simulink model "sim2DOFArmSynergyTemplate"  (R2017a)
settings: Solver=FixedStepAuto  StartTime=0.0  StopTime=6  RelTol=1e-3
undefined symbols (not defined in the file): alpha, armDynamics, get
libraries: vrlib x4, sldrtlib x1
settings Model: Creator=ricardog  LastModifiedBy=ricardog
settings SolverCC: AutoInsertRateTranBlk=on

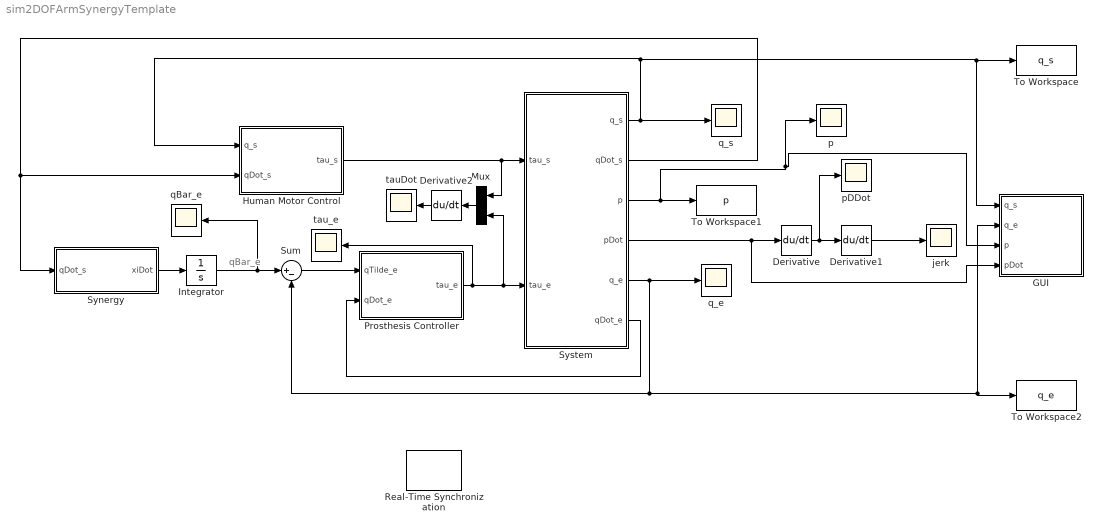
== system sim2DOFArmSynergyTemplate ==
  note: qBar_e
  Derivative : Derivative
  Derivative1 : Derivative
  Derivative2 : Derivative
  GUI : Subsystem
  Human Motor Control : Subsystem
  Integrator : Integrator  InitialCondition=get(armDynamics,'qInit_e')
  Mux : Mux  Inputs=2
  Prosthesis Controller : Subsystem
  Real-Time Synchronization : sldrtlib/Real-Time Synchronization  SampleTime=0.01  MaxMissedTicks=50  ShowMissedTicks=off  YieldWhenWaiting=off
  Sum : Sum  Inputs=|+-
  Synergy : Subsystem
  System : Subsystem
  To Workspace : ToWorkspace  VariableName=q_s  SampleTime=-1
  To Workspace1 : ToWorkspace  VariableName=p  SampleTime=-1
  To Workspace2 : ToWorkspace  VariableName=q_e  SampleTime=-1
  jerk : Scope
  p : Scope
  pDDot : Scope
  qBar_e : Scope
  q_e : Scope
  q_s : Scope
  tauDot : Scope
  tau_e : Scope
  wires:
  Human Motor Control/1(tau_s) -> Mux/1, System/1(tau_s)
  Prosthesis Controller/1(tau_e) -> Mux/2, System/2(tau_e), tau_e/1
  System/6(qDot_e) -> Prosthesis Controller/2(qDot_e)
  System/5(q_e) -> q_e/1, GUI/2(q_e), To Workspace2/1, Sum/2
  Sum/1 -> Prosthesis Controller/1(qTilde_e)
  Synergy/1(xiDot) -> Integrator/1
  Integrator/1 -> qBar_e/1, Sum/1
  System/3(p) -> To Workspace1/1, GUI/3(p), p/1
  System/4(pDot) -> GUI/4(pDot), Derivative/1
  Derivative/1 -> pDDot/1, Derivative1/1
  Derivative1/1 -> jerk/1
  System/2(qDot_s) -> Human Motor Control/2(qDot_s), Synergy/1(qDot_s)
  Derivative2/1 -> tauDot/1
  Mux/1 -> Derivative2/1
  System/1(q_s) -> GUI/1(q_s), To Workspace/1, Human Motor Control/1(q_s), q_s/1

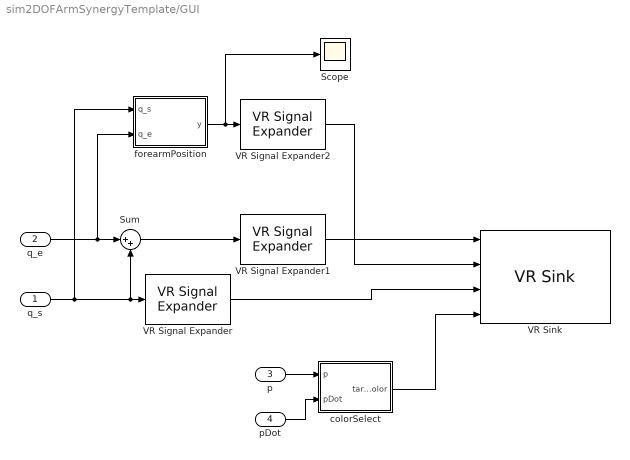
== system sim2DOFArmSynergyTemplate/GUI ==
  q_s : Inport
  q_e : Inport  Port=2
  p : Inport  Port=3
  pDot : Inport  Port=4
  Scope : Scope
  Sum : Sum  Inputs=|++
  VR Signal Expander : vrlib/VR Signal Expander  outwidth=4  outidx=[4]
      settings: SourceProductName=Simulink 3D Animation  SourceProductBaseCode=VR
  VR Signal Expander1 : vrlib/VR Signal Expander  outwidth=4  outidx=[4]
      settings: SourceProductName=Simulink 3D Animation  SourceProductBaseCode=VR
  VR Signal Expander2 : vrlib/VR Signal Expander  outwidth=3  outidx=[1 2]
      settings: SourceProductName=Simulink 3D Animation  SourceProductBaseCode=VR
  VR Sink : vrlib/VR Sink  InstantiateOnLoad=on  SampleTime=0.1  ViewEnable=on  RemoteChange=off  RemoteView=off  FieldsWritten=Forearm.rotation.4.1.1.double#Forearm.translation.3.1.1.double#UpperArm.rotation.4.1.1.double#EndTarget_material.diffuseColor.3.1.1.double  WorldFileName=C:\Users\ricardog\Documents\Workspace\HRSC_FW\GUI\armTargetsGUI.wrl  AutoView=on  VideoDimensions=[]  AllowVariableSize=off  FigureProperties="{'Position', 'Name', 'Viewpoint', 'CameraBound', 'CameraDirection', 'CameraPosition', 'CameraUpVector', 'ZoomFactor', 'Antialiasing', 'Headlight', 'Lighting', 'NavPanel', 'Sound', 'StatusBar', 'Stereo3D', 'Stereo3DCameraOffset', 'Stereo3DHIT', 'ToolBar', 'Textures', 'Transparency', 'Triad', 'Wireframe', 'NavZones', 'NavMode', 'NavSpeed', 'CaptureFileFormat', 'CaptureFileName', 'Record2DCompressMethod', 'Record2DCompressQuality', 'Record2D', 'Record2DFileName', 'Record2DFPS'; [5.8000000000000007e+00   9.1799999999999955e+01   6.8880000000000007e+02   4.7160000000000002e+02], '', 'Side view', 'on', [0.0000000000000000e+00   0.0000000000000000e+00  -1.0000000000000000e+00], [0.0000000000000000e+00   0.0000000000000000e+00   0.0000000000000000e+00], [0.0000000000000000e+00   1.0000000000000000e+00   0.0000000000000000e+00], [1.0000000000000000e+00], 'on', 'on', 'on', 'halfbar', 'on', 'on', 'off', [1.0000000149011612e-01], [0.0000000000000000e+00], 'on', 'on', 'on', 'none', 'off', 'off', 'examine', 'normal', 'tif', '%f_anim_%n.tif', 'auto', [7.5000000000000000e+01], 'off', '%f_anim_%n.avi', 'auto'}"
      settings: SourceProductBaseCode=VR
  colorSelect : MATLAB Function  TreatAsAtomicUnit=on
  forearmPosition : MATLAB Function  TreatAsAtomicUnit=on
  wires:
  q_s/1 -> Sum/2, VR Signal Expander/1, forearmPosition/1(q_s)
  forearmPosition/1(y) -> Scope/1, VR Signal Expander2/1
  Sum/1 -> VR Signal Expander1/1
  q_e/1 -> forearmPosition/2(q_e), Sum/1
  VR Signal Expander1/1 -> VR Sink/1
  VR Signal Expander2/1 -> VR Sink/2
  VR Signal Expander/1 -> VR Sink/3
  p/1 -> colorSelect/1(p)
  pDot/1 -> colorSelect/2(pDot)
  colorSelect/1(targetColor) -> VR Sink/4

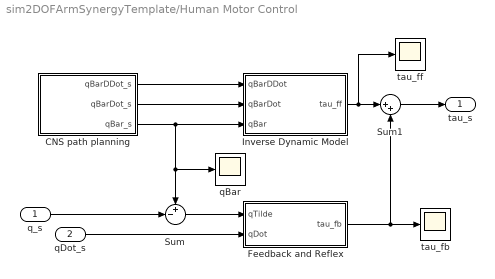
== system sim2DOFArmSynergyTemplate/Human Motor Control ==
  q_s : Inport
  qDot_s : Inport  Port=2
  CNS path planning : Subsystem
  Feedback and Reflex : Subsystem
  Inverse Dynamic Model : Subsystem
  Sum : Sum  Inputs=+-|
  Sum1 : Sum  Inputs=|++
  qBar : Scope
  tau_fb : Scope
  tau_ff : Scope
  tau_s : Outport
  wires:
  CNS path planning/2(qBarDot_s) -> Inverse Dynamic Model/2(qBarDot)
  CNS path planning/1(qBarDDot_s) -> Inverse Dynamic Model/1(qBarDDot)
  CNS path planning/3(qBar_s) -> Inverse Dynamic Model/3(qBar), qBar/1, Sum/1
  q_s/1 -> Sum/2
  qDot_s/1 -> Feedback and Reflex/2(qDot)
  Sum/1 -> Feedback and Reflex/1(qTilde)
  Inverse Dynamic Model/1(tau_ff) -> Sum1/1, tau_ff/1
  Feedback and Reflex/1(tau_fb) -> tau_fb/1, Sum1/2
  Sum1/1 -> tau_s/1

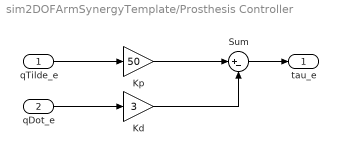
== system sim2DOFArmSynergyTemplate/Prosthesis Controller ==
  qTilde_e : Inport
  qDot_e : Inport  Port=2
  Kd : Gain  Gain=3
  Kp : Gain  Gain=50
  Sum : Sum  Inputs=|+-
  tau_e : Outport
  wires:
  qTilde_e/1 -> Kp/1
  qDot_e/1 -> Kd/1
  Kp/1 -> Sum/1
  Kd/1 -> Sum/2
  Sum/1 -> tau_e/1

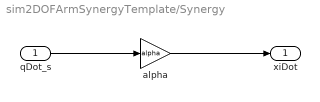
== system sim2DOFArmSynergyTemplate/Synergy ==
  qDot_s : Inport
  alpha : Gain  Gain=alpha
  xiDot : Outport
  wires:
  qDot_s/1 -> alpha/1
  alpha/1 -> xiDot/1

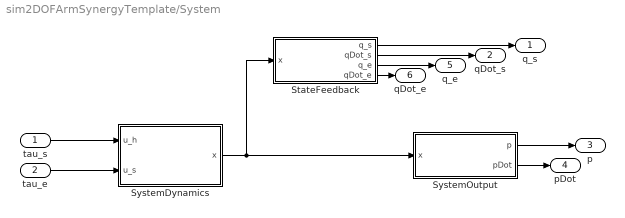
== system sim2DOFArmSynergyTemplate/System ==
  tau_s : Inport
  tau_e : Inport  Port=2
  StateFeedback : Subsystem
  SystemDynamics : Subsystem
  SystemOutput : Subsystem
  q_s : Outport
  qDot_s : Outport  Port=2
  p : Outport  Port=3
  pDot : Outport  Port=4
  q_e : Outport  Port=5
  qDot_e : Outport  Port=6
  wires:
  SystemDynamics/1(x) -> StateFeedback/1(x), SystemOutput/1(x)
  SystemOutput/1(p) -> p/1
  tau_s/1 -> SystemDynamics/1(u_h)
  tau_e/1 -> SystemDynamics/2(u_s)
  SystemOutput/2(pDot) -> pDot/1
  StateFeedback/1(q_s) -> q_s/1
  StateFeedback/3(q_e) -> q_e/1
  StateFeedback/2(qDot_s) -> qDot_s/1
  StateFeedback/4(qDot_e) -> qDot_e/1

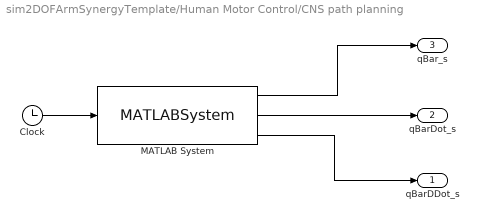
== system sim2DOFArmSynergyTemplate/Human Motor Control/CNS path planning ==
  Clock : Clock
  MATLAB System : MATLABSystem  System=trajGen  q_o=get(armDynamics,'qInit_s')  qDot_o=0  qDDot_o=0  q_f=pi/3  qDot_f=0  qDDot_f=0  t_o=1  t_f=4  d_max=0  SimulateUsing=Interpreted execution
      mask Type: trajGen
      mask Display:
      | disp('trajGen');
      | port_label('input',1,'t');
      | port_label('output',1,'qBar');
      | port_label('output',2,'qBarDot');
      | port_label('output',3,'qBarDDot');
  qBarDDot_s : Outport
  qBarDot_s : Outport  Port=2
  qBar_s : Outport  Port=3
  wires:
  MATLAB System/2 -> qBarDot_s/1
  MATLAB System/3 -> qBarDDot_s/1
  Clock/1 -> MATLAB System/1
  MATLAB System/1 -> qBar_s/1

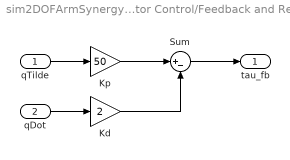
== system sim2DOFArmSynergyTemplate/Human Motor Control/Feedback and Reflex ==
  qTilde : Inport
  qDot : Inport  Port=2
  Kd : Gain  Gain=2
  Kp : Gain  Gain=50
  Sum : Sum  Inputs=|+-
  tau_fb : Outport
  wires:
  qTilde/1 -> Kp/1
  Kp/1 -> Sum/1
  qDot/1 -> Kd/1
  Kd/1 -> Sum/2
  Sum/1 -> tau_fb/1

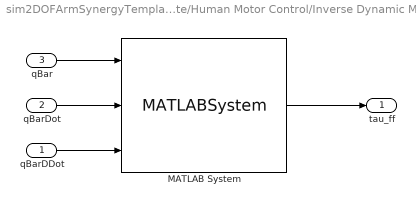
== system sim2DOFArmSynergyTemplate/Human Motor Control/Inverse Dynamic Model ==
  qBarDDot : Inport
  qBarDot : Inport  Port=2
  qBar : Inport  Port=3
  MATLAB System : MATLABSystem  System=hmcIDM  kS=0  kE=0  dS=-1.0  dE=-1.0  lA=0.29  lF=0.32  mA=1.93  mF=1.52  q0=0  SimulateUsing=Code generation
      mask Type: hmcIDM
      mask Display:
      | disp('hmcIDM');
      | port_label('input',1,'qBar');
      | port_label('input',2,'qBarDot');
      | port_label('input',3,'qBarDDot');
      | port_label('output',1,'tau');
  tau_ff : Outport
  wires:
  qBar/1 -> MATLAB System/1
  qBarDot/1 -> MATLAB System/2
  qBarDDot/1 -> MATLAB System/3
  MATLAB System/1 -> tau_ff/1

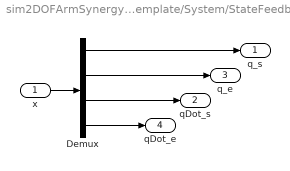
== system sim2DOFArmSynergyTemplate/System/StateFeedback ==
  x : Inport
  Demux : Demux
  q_s : Outport
  qDot_s : Outport  Port=2
  q_e : Outport  Port=3
  qDot_e : Outport  Port=4
  wires:
  x/1 -> Demux/1
  Demux/1 -> q_s/1
  Demux/3 -> qDot_s/1
  Demux/4 -> qDot_e/1
  Demux/2 -> q_e/1

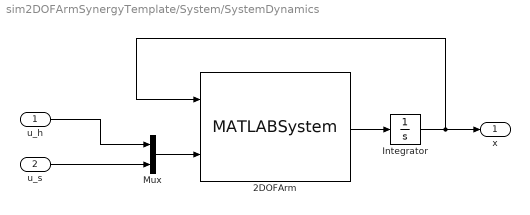
== system sim2DOFArmSynergyTemplate/System/SystemDynamics ==
  u_h : Inport
  u_s : Inport  Port=2
  2DOFArm : MATLABSystem  System=armDynamics  kS=0  kE=0  dS=-1.2  dE=-1.2  lA=0.31  lF=0.34  mA=1.93  mF=1.52  q0=[ 0; pi/2 ]  qInit_s=pi/8  qInit_e=7*pi/8  qInit=[ pi/8; 7*pi/8 ]  qDotInit=[ 0; 0 ]  SimulateUsing=Code generation
      mask Type: armDynamics
      mask Display:
      | disp('armDynamics');
      | port_label('input',1,'x');
      | port_label('input',2,'u');
      | port_label('output',1,'xDot');
  Integrator : Integrator  InitialCondition=[get(armDynamics,'qInit');get(armDynamics,'qDotInit')]  UpperSaturationLimit=100  LowerSaturationLimit=-100
  Mux : Mux  Inputs=2
  x : Outport
  wires:
  Mux/1 -> 2DOFArm/2
  u_h/1 -> Mux/1
  u_s/1 -> Mux/2
  2DOFArm/1 -> Integrator/1
  Integrator/1 -> 2DOFArm/1, x/1

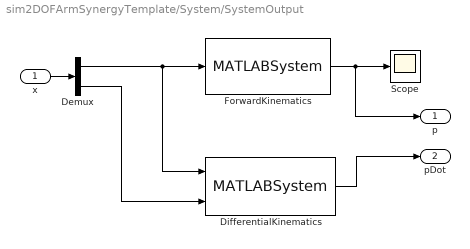
== system sim2DOFArmSynergyTemplate/System/SystemOutput ==
  x : Inport
  Demux : Demux  Outputs=2
  DifferentialKinematics : MATLABSystem  System=armDiffK  SimulateUsing=Code generation
      mask Type: armDiffK
      mask Display:
      | disp('armDiffK');
      | port_label('input',1,'q');
      | port_label('input',2,'qDot');
      | port_label('output',1,'vHand');
  ForwardKinematics : MATLABSystem  System=armFK  SimulateUsing=Code generation
      mask Type: armFK
      mask Display:
      | disp('armFK');
      | port_label('input',1,'q');
      | port_label('output',1,'xHand');
  Scope : Scope
  p : Outport
  pDot : Outport  Port=2
  wires:
  x/1 -> Demux/1
  Demux/1 -> DifferentialKinematics/1, ForwardKinematics/1
  Demux/2 -> DifferentialKinematics/2
  DifferentialKinematics/1 -> pDot/1
  ForwardKinematics/1 -> p/1, Scope/1

== matlab function sim2DOFArmSynergyTemplate/GUI/colorSelect ==
  data: p input; targetColor output; pDot input
function targetColor = fcn(p,pDot)
p_f = [0.5969;-0.0670];   % Desired end position
pNorm = norm(p-p_f);
pDotNorm = norm(pDot);
if(pNorm<0.01 && pDotNorm<0.1)
    R = 0;
    G = 1;
    B = 0;
else
    R = 0;
    G = 0;
    B = 1;
end
targetColor = [R;G;B];

== matlab function sim2DOFArmSynergyTemplate/GUI/forearmPosition ==
  data: q_s input; y output; q_e input
function y = fcn(q_s,q_e)
lA = get(armDynamics,'lA');
lF = get(armDynamics,'lF');
% xArm = (lA+(1/2)*lF)*sin(q);
% yArm = -(lA+(1/2)*lF)*cos(q);
xArm = lA*sin(q_s)+(1/2)*lF*sin(q_s+q_e);
yArm = -lA*cos(q_s)-(1/2)*lF*cos(q_s+q_e);
% xArm = lA*sin(q_s);
% yArm = -lA*cos(q_s);
% xArm = 0;
% yArm = 0;
y = [xArm;yArm];
